simulink model "SSN2"  (Simulink 7.6)
settings: Solver=FixedStepDiscrete  StartTime=0.0  StopTime=10.0  FixedStep=0.5  RelTol=1e-3
libraries: xpclib x1
(part 3 of 3)

== matlab function Linear Feedback/Embedded Kalman Decode/linear ==
  data: ws1 input double; Gain input double; Jbias input double; DECVECS input double; ENCVECS input double; seed input double; neural input double; x0 input double; out output double; DFm input double; Sm input double
function out = SSN(ws1, Gain, Jbias, DECVECS, ENCVECS, seed, neural, x0, DFm, Sm)
% Setup a Kalman-filter decoder.

%% INITIALIZE PARAMETERS
% There are the same for all the simulation and should be set only once
binsize = 0.050; %bin for the neural recording
dt      = 0.001; %simulation time constant         

N       = 1000;
%assert(N == ws1);
NumEns  = 2;
      
persistent tauPSC           
persistent TimeConstant              
persistent tref             
persistent trc              
persistent epsSoma

if isempty(binsize) || isempty(tauPSC)||isempty(TimeConstant) || isempty(dt) || isempty(tref)||isempty(trc) ||isempty(epsSoma)
    
    tauPSC           = 0.02;  %post-synaptic current time constant
    TimeConstant     = 0.005; %filter time constant
    tref             = 0.001; %refractory period of neurons
    trc              = 0.02;  %RC time constant of neurons
    epsSoma          = dt/trc;
end
    
% Encoding and Decoding vectors.
persistent In_Start
persistent Out_Start

if isempty(In_Start) || isempty(Out_Start)
    In_Start    = 1:NumEns;
    Out_Start   = 1:NumEns;
end

%% SET UP CONNECTION MATRICES

persistent Mxd
persistent Myd

% Make the matrices neurally plausible
if isempty(Mxd) || isempty(Myd)
    Matrix_X = zeros(3,3);
    Matrix_X(1:2, 1:2) = DFm(4:5, 4:5);
    Matrix_X(1:2, 3) = DFm(4:5, 7);
    Matrix_X(3, 3) = DFm(7, 7);
    
    Matrix_Y = zeros(3,96);
    Matrix_Y(1:2,:) = Sm(4:5,:);
    Matrix_Y(3,:) = Sm(7,:);

    % Go from discret time to continuous time
    Mxc = (Matrix_X-eye(size(Matrix_X)))/binsize;
    Myc = Matrix_Y/binsize;
    % Go from continuous time to discrete synapse
    Mxd = tauPSC*Mxc+eye(size(Matrix_X));
    Myd = tauPSC*Myc;
end

% Setup coupling matrices in local variables
persistent CMatrix
persistent FilMatrix

if isempty(CMatrix) || isempty(FilMatrix) 
    
    M         = Mxd(1:2,1:2);
    CMatrix   = zeros(NumEns,NumEns,NumEns);
    FilMatrix = zeros(NumEns,NumEns);
    
    for m=1:NumEns
        for n=1:NumEns
            mi               = In_Start(m);
            ni               = In_Start(n);
            SynA             = dt/tauPSC;
            CMatrix(mi,ni,n) = (SynA)* M(m,n);
            FilMatrix(mi,n)  = (1-SynA);
        end
    end
end

persistent xk;
if seed == 1 || isempty(xk)
    % initialize
    xk = x0(4:5,1);
    
    % handle initial condition
    out = xk;
else
    

%% RUN SIMULATION
% Perform simulation at each time step
for ii = 1:binsize/dt
    xk = (runsimulation(N, tref, TimeConstant, dt, Mxd, Myd, NumEns, Gain, Jbias, epsSoma, In_Start, DECVECS, ENCVECS, CMatrix, FilMatrix, Out_Start, neural))';
    out = xk;
end

end
%% RUN THE SIMULATION
function runDatanetwork = runsimulation(N, tref, TimeConstant, dt, Mxd, Myd, NumEns, Gain, Jbias, epsSoma, In_Start, DECVECS, ENCVECS, CMatrix, FilMatrix, Out_Start, Neuralspikes)

% Set the inputs signals
ext_INPUTS = Myd(1:2,:) * Neuralspikes + Mxd(1:2, 3);

% Set up the storage and initialize arrays

% Storage for ensemble variables
persistent Vsoma;
persistent InRef;

if isempty(Vsoma) || isempty(InRef)
    Vsoma   = zeros(N, NumEns);
    InRef   = zeros(N, NumEns);
    
    for m=1:NumEns
        Vsoma(:, m) = rand(N,1);
        InRef(:, m) = zeros(N,1);
    end
end

% Initialize storage for output data
persistent sys_OUTPUTS;

if isempty(sys_OUTPUTS)
    sys_OUTPUTS = zeros(1,NumEns);
end

% Initialize storage for state vectors data
persistent vectorValue; %% Holds all the system state vectors.
persistent newValues;   %% Holds all the temporary system state vectors.
persistent filterTmp;   %% Intermediate storage for the filters.

if isempty(vectorValue) || isempty(newValues) || isempty(filterTmp)
    vectorValue = zeros(NumEns, 1);    
    newValues   = zeros(NumEns, NumEns);
    filterTmp   = zeros(NumEns, NumEns);
end

%%%%%%%%%%%%%%%%%%%%%%%%%%%%%%%%%%%%%%%%
%%%% RUN THE SIMULATION %%%%%%%%%%%%%%%%
%%%%%%%%%%%%%%%%%%%%%%%%%%%%%%%%%%%%%%%%

% Update and filter the inputs to the neurons
for n=1:NumEns
    ni = In_Start(n);
    newValues(:,n) = CMatrix(:,ni,n)*vectorValue(ni);
    filterTmp(:,n) = FilMatrix(:,n).*filterTmp(:,n)+newValues(:,n);
end

vectorValue = sum(filterTmp(1:NumEns,:),2);

% Add in the external input signals
for m=1:NumEns
    mi              = In_Start(m);
    vectorValue(mi) = vectorValue(mi) + ext_INPUTS(m,1); 
end

% Pass the state vector through the neuronal nonlinearity and compute the
% estimated state vector values
for m=1:NumEns
    sysIndex   = In_Start(m);
    
    J                  = Jbias(:, m) + Gain(:, m).*(vectorValue(sysIndex)'*ENCVECS(sysIndex,1:N))';
    V                  = Vsoma(:, m);
    inref              = InRef(:, m);
    
    dV                 = epsSoma*(J-V); % RC exponential increase
    V                  = V+dV;
    
    output             = zeros(N,1);
    for ii = 1: length(V)
        if V(ii)>1
            deltaT     = dt*(V(ii)-1)./dV(ii); % Interpolated spike time
            output(ii) = 1/dt;
            inref(ii)  = tref+dt-deltaT;      % We subtract dt in the next loop
        end
    end
    
    for ii = 1: length(inref)
        if inref(ii)>0
            V(ii)     = 0.0;                   % Reset the soma to 0 for neurons in refractory period.
            inref(ii) = inref(ii) - dt;     % Countdown
            if inref(ii)<=0
                V(ii) = epsSoma*J(ii).*(-inref(ii)/dt);
            end
        end
    end
    
%    spikeIndex         = find(V>1);                            % Normalized threshold = 1
%     deltaT             = dt*(V(spikeIndex)-1)./dV(spikeIndex); % Interpolated spike time
%     output             = zeros(N,1);
%     output(spikeIndex) = 1/dt;      
%     
%     inref(spikeIndex)  = tref+dt-deltaT;      % We subtract dt in the next loop
%     itest              = find(inref>0);       % Neurons in refractory period
%     if(~isempty(itest))
%         V(itest)     = 0.0;                   % Reset the soma to 0 for neurons in refractory period.
%         inref(itest) = inref(itest) - dt;     % Countdown
%         i2           = find(inref(itest)<=0); % Find those out of the refractory period
%         if(~isempty(i2))                      % Interpolate the voltage for the time out of the refractory period.
%             itest2    = itest(i2);
%             V(itest2) = epsSoma*J(itest2).*(-inref(itest2)/dt);
%         end
%     end
    V                           = (V>0).*V;
    Vsoma(:, m)                 = V;                      % Save tmp values in cells
    InRef(:, m)                 = inref;
    vectorValue(sysIndex)       = DECVECS(sysIndex,1:N)*output;
    
    sys_OUTPUTS(1,Out_Start(m)) = vectorValue(sysIndex)'; % Save the present (unfiltered) values of state vectors
end

% Save precedent signal for filtering
persistent pastsignal;

if isempty(pastsignal)
    pastsignal = zeros(1,2);
end

% Data to output
runDatanetwork = zeros(1,2);

% Filter the output
for n=1:NumEns
    runDatanetwork(1,n) = FilterSignal(pastsignal(1,n), sys_OUTPUTS(1,n), dt, TimeConstant);
end

% Save precedent signal for filtering
pastsignal = runDatanetwork;

% Function to perform the filtering
function FilSignal = FilterSignal(pastSignal, newSignal, dt, TimeConstant)
    if TimeConstant == 0
        FilSignal = newSignal(:, end);
    else
        if(TimeConstant<dt)
            eps = 1;
        else
            eps = dt/TimeConstant;
        end
        FilSignal = (1-eps)*pastSignal+eps*newSignal;
    end
